simulink model "part1_1"  (R2018b)
settings: Solver=VariableStepAuto  StartTime=0.0  StopTime=2  RelTol=1e-3
settings Model: Creator=lisazaher  LastModifiedBy=lisazaher

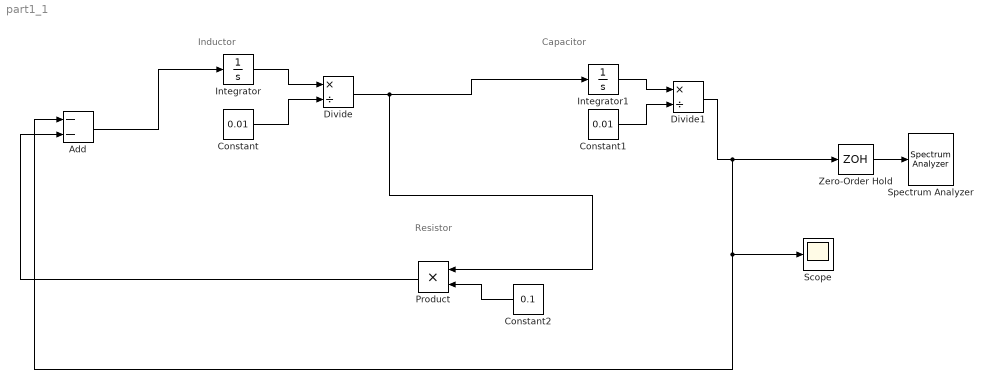
== system part1_1 ==
  note: Resistor
  note: Capacitor
  note: Inductor
  Add : Sum  Inputs=--
  Constant : Constant  Value=0.01
  Constant1 : Constant  Value=0.01
  Constant2 : Constant  Value=0.1
  Divide : Product  Inputs=*/
  Divide1 : Product  Inputs=*/
  Integrator : Integrator  InitialCondition=0.1
  Integrator1 : Integrator  InitialCondition=0.1
  Product : Product
  Scope : Scope
  Spectrum Analyzer : SpectrumAnalyzer
  Zero-Order Hold : ZeroOrderHold  SampleTime=2^-10
  wires:
  Integrator/1 -> Divide/1
  Constant/1 -> Divide/2
  Integrator1/1 -> Divide1/1
  Constant1/1 -> Divide1/2
  Divide/1 -> Product/1, Integrator1/1
  Constant2/1 -> Product/2
  Product/1 -> Add/2
  Divide1/1 -> Zero-Order Hold/1, Scope/1, Add/1
  Add/1 -> Integrator/1
  Zero-Order Hold/1 -> Spectrum Analyzer/1
